simulink model "NonlinearSim2"  (R2020a)
settings: Solver=ode45  StartTime=0.0  StopTime=20  FixedStep=1e-3  RelTol=1e-3  EnableMultiTasking=on
values from neighbouring files (symbols this model uses):
  b = 0.05    [Main.m]
  m = 0.25    [Main.m]
  M = 1.0    (= 1)    [Main.m]
libraries: cstblocks x2
settings Model: Creator=FawaD KhaN  LastModifiedBy=FawaD KhaN
settings DataIOCC: LimitDataPoints=on  SaveFormat=Array  ReturnWorkspaceOutputs=off
settings OptimizationCC: LifeSpan=inf
settings DebuggingCC: SFUnexpectedBacktrackingDiag=warning  SFNoUnconditionalDefaultTransitionDiag=warning  SFExecutionAtInitializationDiag=none  ArithmeticOperatorsInVariantConditions=warning
settings HardwareCC: ProdBitPerPointer=32  ProdBitPerSizeT=32  ProdBitPerPtrDiffT=32  ProdLargestAtomicFloat=None  ProdIntDivRoundTo=Undefined  ProdEndianess=Unspecified  ProdWordSize=32  ProdHWDeviceType=32-bit Generic
settings ModelReferenceCC: PropagateSignalLabelsOutOfModel=off
settings SFSimCC: SimUseLocalCustomCode=off  CustomCodeUndefinedFunction=UseInterfaceOnly
settings RTWCC: RTWUseLocalCustomCode=off
settings CodeAppCC: StateflowObjectComments=on
settings GRTTargetCC: TargetLangStandard=C89/C90 (ANSI)
settings ConfigComp: CovMetricSettings=dw  CovHtmlReporting=on  CovSaveCumulativeToWorkspaceVar=on  CovSaveSingleToWorkspaceVar=on  CovExternalEMLEnable=off

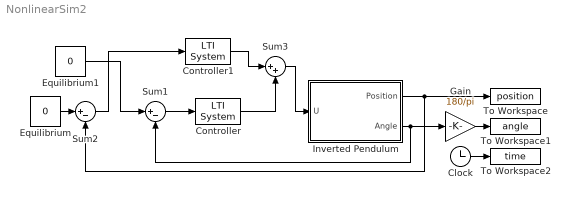
== system NonlinearSim2 ==
  Clock : Clock
  Controller : cstblocks/LTI System  sys=K  IC=[]
  Controller1 : cstblocks/LTI System  sys=K2  IC=[]
  Equilibrium : Constant  Value=0
  Equilibrium1 : Constant  Value=0
  Gain : Gain  Gain=180/pi
  Inverted Pendulum : Subsystem
  Sum1 : Sum  Inputs=|+-
  Sum2 : Sum  Inputs=|+-
  Sum3 : Sum  Inputs=|++
  To Workspace : ToWorkspace  VariableName=position  SampleTime=-1
  To Workspace1 : ToWorkspace  VariableName=angle  SampleTime=-1
  To Workspace2 : ToWorkspace  VariableName=time  SampleTime=-1
  wires:
  Gain/1 -> To Workspace1/1
  Sum1/1 -> Controller/1
  Equilibrium1/1 -> Sum1/1
  Sum2/1 -> Controller1/1
  Equilibrium/1 -> Sum2/1
  Controller/1 -> Sum3/2
  Clock/1 -> To Workspace2/1
  Inverted Pendulum/2(Angle) -> Gain/1, Sum1/2
  Inverted Pendulum/1(Position) -> To Workspace/1, Sum2/2
  Controller1/1 -> Sum3/1
  Sum3/1 -> Inverted Pendulum/1(U)

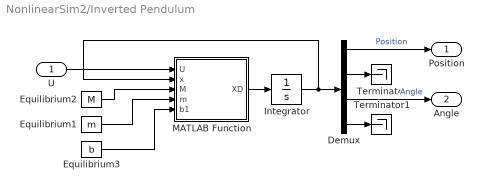
== system NonlinearSim2/Inverted Pendulum ==
  U : Inport
  Demux : Demux
  Equilibrium1 : Constant  Value=m
  Equilibrium2 : Constant  Value=M
  Equilibrium3 : Constant  Value=b
  Integrator : Integrator  InitialCondition=[0;0;pi/3;0]
  MATLAB Function : MATLAB Function  TreatAsAtomicUnit=on
  Terminator : Terminator
  Terminator1 : Terminator
  Position : Outport
  Angle : Outport  Port=2
  wires:
  Equilibrium2/1 -> MATLAB Function/3(M)
  MATLAB Function/1(XD) -> Integrator/1
  U/1 -> MATLAB Function/1(U)
  Equilibrium1/1 -> MATLAB Function/4(m)
  Demux/3 -> Angle/1  "Angle"
  Demux/1 -> Position/1  "Position"
  Demux/2 -> Terminator/1
  Demux/4 -> Terminator1/1
  Integrator/1 -> Demux/1, MATLAB Function/2(x)
  Equilibrium3/1 -> MATLAB Function/5(b1)

== matlab function NonlinearSim2/Inverted Pendulum/MATLAB Function ==
  data: U input; XD output; x input; M input; m input; b1 input
function XD = fcn(U,x,M,m,b1)
l  = 0.5;
b1 = 0.05;
g  = 9.81;

%% assign states
y  = x(1);
dy = x(2);
theta  = x(3);
dtheta = x(4);

%% assign inputs
F = U(1);
%% Compute Derivatives
ydot     = dy;
thetadot = dtheta;

M = [M+m, m*(l/2)*cos(theta);...
     m*(l/2)*cos(theta), m*(l^2)/4];
 
c = [m*(l/2)*thetadot^2*sin(theta) + F - b1*ydot;...
     m*g*(l/2)*sin(theta)];
 
tmp = M\c;

yddot = tmp(1);
thetaddot = tmp(2);
n = [ydot;yddot];
q = [thetadot;thetaddot];

XD = [n;q];
